simulink model "pendulum"  (R2018b)
settings: Solver=ode1  StartTime=0.0  StopTime=40  FixedStep=.001  RelTol=1e-3
values from neighbouring files (symbols this model uses):
  A = [0 0 0 -10 1 0 0 -1 0 1 0 -2 ... (16 elements, 4x4)]    [final2 FUNCIONA.mat]    (also in funcionaobservador.mat)
  B = [0 0 0 1]    [final2 FUNCIONA.mat]    (also in funcionaobservador.mat)
  C = [13 7 0 0]    [final2 FUNCIONA.mat]    (also in funcionaobservador.mat)
  C2 = [1 0 0 -1]    [final2 FUNCIONA.mat]    (also in funcionaobservador.mat)
  K = [110 153 69 11]    [final2 FUNCIONA.mat]    (also in funcionaobservador.mat)
settings Model: Creator=Abraham Pérez  LastModifiedBy=Abraham Pérez
settings SolverCC: InitialStep=.001  ZeroCrossAlgorithm=Adaptive
settings DebuggingCC: IgnoredZcDiagnostic=none

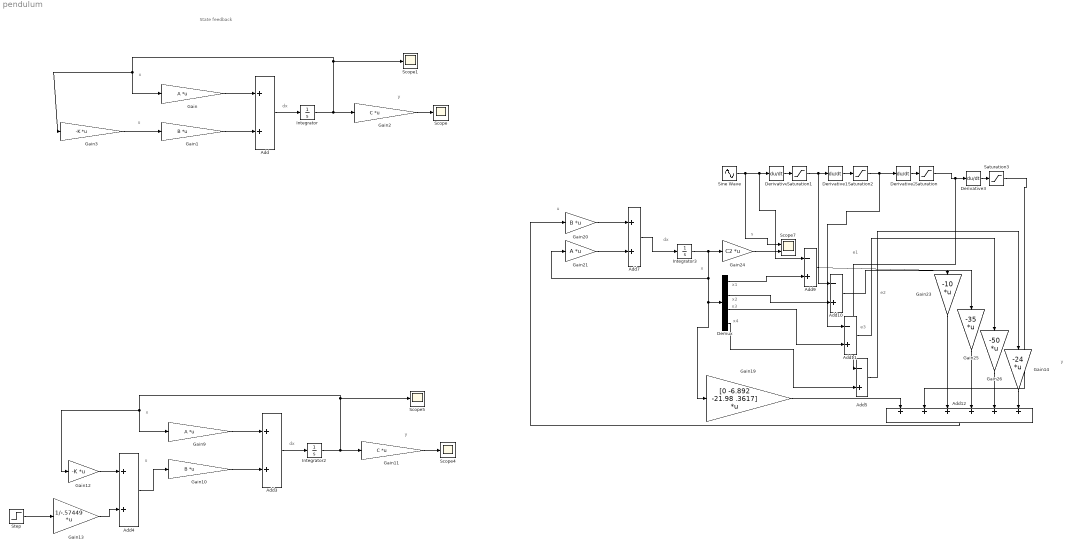
== system pendulum ==
  note: x4
  note: State feedback
  note: y
  note: dx
  note: u
  note: x
  note: dx
  note: x
  note: y
  note: u
  note: y
  note: e3
  note: x
  note: s
  note: e2
  note: x1
  note: x3
  note: dx
  note: u
  note: x2
  note: e1
  Add{,3..4,7} (4 alike) : Sum
  Add{5,9..11} (4 alike) : Sum  Inputs=-+
  Add12 : Sum  Inputs=++++++
  Demux : Demux
  Derivative{,1..3} (4 alike) : Derivative
  Gain : Gain  Gain=A  Multiplication=Matrix(K*u)
  Gain1 : Gain  Gain=B  Multiplication=Matrix(K*u)
  Gain10 : Gain  Gain=B  Multiplication=Matrix(K*u)
  Gain11 : Gain  Gain=C  Multiplication=Matrix(K*u)
  Gain12 : Gain  Gain=-K  Multiplication=Matrix(K*u)
  Gain13 : Gain  Gain=1/-.57449  Multiplication=Matrix(K*u)
  Gain14 : Gain  Gain=-24  Multiplication=Matrix(K*u)
  Gain19 : Gain  Gain=[0 -6.892 -21.98 .3617]  Multiplication=Matrix(K*u)
  Gain2 : Gain  Gain=C  Multiplication=Matrix(K*u)
  Gain20 : Gain  Gain=B  Multiplication=Matrix(K*u)
  Gain21 : Gain  Gain=A  Multiplication=Matrix(K*u)
  Gain23 : Gain  Gain=-10  Multiplication=Matrix(K*u)
  Gain24 : Gain  Gain=C2  Multiplication=Matrix(K*u)
  Gain25 : Gain  Gain=-35  Multiplication=Matrix(K*u)
  Gain26 : Gain  Gain=-50  Multiplication=Matrix(K*u)
  Gain3 : Gain  Gain=-K  Multiplication=Matrix(K*u)
  Gain9 : Gain  Gain=A  Multiplication=Matrix(K*u)
  Integrator : Integrator  InitialCondition=[-1 .5 .5 1]
  Integrator2 : Integrator  InitialCondition=[-1 .5 .5 1]
  Integrator3 : Integrator  InitialCondition=[1 .5 .5 1]
  Saturation{,1..3} (4 alike) : Saturate  UpperLimit=1  LowerLimit=-1
  Scope{,1,4..5} (4 alike) : Scope
  Scope7 : Scope  NumInputPorts=2
  Sine Wave : Sin  Amplitude=.05  SampleTime=0
  Step : Step  After=26  SampleTime=0
  wires:
  Integrator/1 -> Gain2/1, Scope1/1, Gain/1, Gain3/1
  Gain/1 -> Add/1
  Gain1/1 -> Add/2
  Add/1 -> Integrator/1
  Gain2/1 -> Scope/1
  Gain3/1 -> Gain1/1
  Step/1 -> Gain13/1
  Gain12/1 -> Add4/1
  Gain13/1 -> Add4/2
  Add4/1 -> Gain10/1
  Gain10/1 -> Add3/2
  Gain11/1 -> Scope4/1
  Gain9/1 -> Add3/1
  Add3/1 -> Integrator2/1
  Integrator2/1 -> Gain11/1, Scope5/1, Gain9/1, Gain12/1
  Integrator3/1 -> Gain19/1, Demux/1, Gain21/1, Gain24/1
  Add11/1 -> Gain26/1
  Add9/1 -> Gain23/1
  Add10/1 -> Gain25/1
  Gain19/1 -> Add12/1
  Gain20/1 -> Add7/1
  Derivative2/1 -> Saturation/1
  Saturation2/1 -> Add11/1, Derivative2/1
  Gain23/1 -> Add12/3
  Gain25/1 -> Add12/4
  Add7/1 -> Integrator3/1
  Saturation1/1 -> Add10/1, Derivative1/1
  Add12/1 -> Gain20/1
  Gain21/1 -> Add7/2
  Derivative/1 -> Saturation1/1
  Saturation/1 -> Add5/1, Derivative3/1
  Gain26/1 -> Add12/5
  Derivative1/1 -> Saturation2/1
  Sine Wave/1 -> Derivative/1, Add9/1, Scope7/1
  Derivative3/1 -> Saturation3/1
  Gain14/1 -> Add12/6
  Add5/1 -> Gain14/1
  Saturation3/1 -> Add12/2
  Demux/1 -> Add9/2
  Demux/2 -> Add10/2
  Demux/3 -> Add11/2
  Demux/4 -> Add5/2
  Gain24/1 -> Scope7/2
